simulink model "Simulink_Pendulum_Control_2019"  (R2019b)
settings: Solver=ode1  StartTime=0.0  StopTime=inf  FixedStep=0.002  RelTol=1e-3  EnableMultiTasking=on
PostLoadFcn:
  | qc_set_target_type(getConfigSet(bdroot, 'QUARC Default Target Configuration'));
values from neighbouring files (symbols this model uses):
  alpha_max = 15    [PolePlacement.m]
  theta_max = 45    [PolePlacement.m]
  voltage_max = 6    [PolePlacement.m]
undefined symbols (not defined in the file or in its folder): A_ob, B_ob, C_ob, D_ob, HIL, Ken_eta, Ken_x, qc_get_step_size, x0_ob
libraries: quarc_library x4, simulink_extras x1
settings Model: SimulationMode=external  ExtModeTrigDuration=5000  Creator=CFulford  LastModifiedBy=federicocorso
settings SolverCC: PositivePriorityOrder=on
settings DataIOCC: LimitDataPoints=on  SaveFormat=Array  SignalLoggingSaveFormat=ModelDataLogs  ReturnWorkspaceOutputs=off
settings OptimizationCC: ExpressionDepthLimit=2147483647  InitFltsAndDblsToZero=on  LifeSpan=inf
settings DebuggingCC: SaveWithParameterizedLinksMsg=none  UnderspecifiedInitializationDetection=Classic  MergeDetectMultiDrivingBlocksExec=none  SolverPrmCheckMsg=warning  MultiTaskDSMMsg=warning  MultiTaskCondExecSysMsg=none  FcnCallInpInsideContextMsg=warning  StateNameClashWarn=warning  SFUnexpectedBacktrackingDiag=warning  SFNoUnconditionalDefaultTransitionDiag=warning  SFExecutionAtInitializationDiag=none  ArithmeticOperatorsInVariantConditions=warning
settings HardwareCC: ProdBitPerPointer=32  ProdBitPerSizeT=32  ProdBitPerPtrDiffT=32  ProdLargestAtomicFloat=None  ProdIntDivRoundTo=Undefined  ProdEndianess=Unspecified  ProdWordSize=32  ProdHWDeviceType=32-bit Generic
settings ModelReferenceCC: PropagateSignalLabelsOutOfModel=off
settings SFSimCC: SimUseLocalCustomCode=off  CustomCodeUndefinedFunction=UseInterfaceOnly
settings RTWCC: Description=QUARC Win64 Target  SystemTargetFile=quarc_win64.tlc  TemplateMakefile=quarc_default_tmf  RTWUseLocalCustomCode=off
settings CodeAppCC: StateflowObjectComments=on
settings STFCustomTargetCC: TargetPreCompLibLocation=C:\PROGRA~3\QUARC\lib\2019b\win64\release  ConcurrentExecutionCompliant=on  CombineOutputUpdateFcns=on  CPPClassGenCompliant=on  SystemTargetFile=quarc_win64.tlc
settings GRTTargetCC: TargetPreCompLibLocation=C:\PROGRA~3\QUARC\lib\2019b\win64\release  TargetLangStandard=C89/C90 (ANSI)  ParMdlRefBuildCompliant=off  CompOptLevelCompliant=off  MatFileLogging=off  UseToolchainInfoCompliant=off  ExtMode=on  ExtModeMexFile=quarc_comm
settings ConfigComp: CovMetricSettings=dw  CovSaveCumulativeToWorkspaceVar=on  CovSaveSingleToWorkspaceVar=on  CovExternalEMLEnable=off  CovSFcnEnable=off

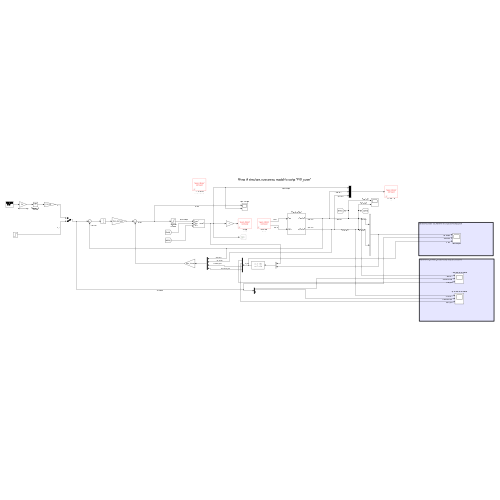
[thumbnail: Simulink's stored preview of the top-level diagram]
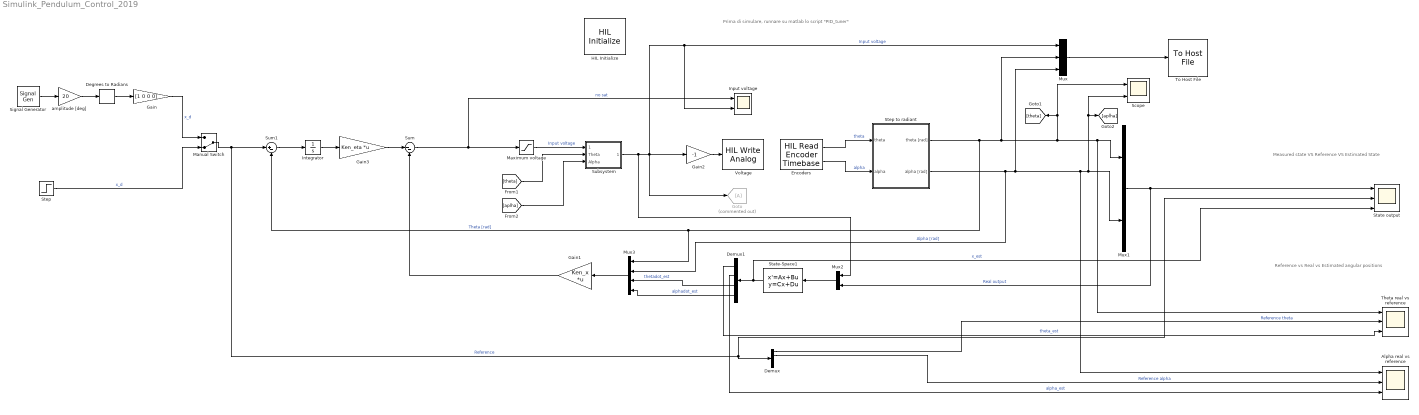
== system Simulink_Pendulum_Control_2019 ==
  note: Measured state VS Reference VS Estimated State
  note: Reference vs Real vs Estimated angular positions
  note: Prima di simulare, runnare su matlab lo script "PID_tuner"
  Alpha real vs reference : Scope  NumInputPorts=3
  Degrees to Radians : simulink_extras/Transformations/Degrees to Radians
  Demux : Demux
  Demux1 : Demux
  Encoders : quarc_library/Data Acquisition/Generic/Timebases/HIL Read Encoder Timebase  object_name=HIL-1  clock=0  channels=[0:1]  samples_in_buffer=max(ceil(1/qc_get_step_size), 1)  active=on  vector_output=off  data_type_mode=Inherit via back propagation  data_type=double
  Gain : Gain  Gain=[1 0 0 0]
  Gain1 : Gain  Gain=Ken_x  Multiplication=Matrix(K*u) (u vector)
  Gain2 : Gain  Gain=-1
  Gain3 : Gain  Gain=Ken_eta  Multiplication=Matrix(K*u) (u vector)
  Goto : Goto  Commented=on
  HIL Initialize : quarc_library/Data Acquisition/Generic/Configuration/HIL Initialize  Priority=-99  object_name=HIL-1  board_type=q2_usb  board_number=0  board_options=d0=digital;d1=digital;led=auto;update_rate=normal;decimation=1  exclusive=off  active=off  hardware_clocks=[0]  clock_modes=[]  initial_clock_frequencies=[]  set_clock_params_at_start=off  set_clock_params_at_switch_in=off  set_clock_frequencies_at_start=off  set_clock_frequencies_at_switch_in=off  analog_input_channels=[0:1]  analog_input_configurations=[]  analog_input_maximums=10  analog_input_minimums=-10  set_analog_input_params_at_start=on  set_analog_input_params_at_switch_in=off  analog_output_channels=[0:1]  analog_output_maximums=10  analog_output_minimums=-10  initial_analog_outputs=[0]  final_analog_outputs=[0]  watchdog_analog_outputs=0  set_analog_output_params_at_start=on  set_analog_output_params_at_switch_in=off  set_analog_outputs_at_start=on  set_analog_outputs_at_switch_in=off  set_analog_outputs_at_terminate=on  set_analog_outputs_at_switch_out=off  set_analog_outputs_on_watchdog=off  digital_input_channels=[]  digital_output_channels=[]  digital_output_configuration=[]  initial_digital_outputs=[1]  final_digital_outputs=[1]  watchdog_digital_outputs=[1]  set_digital_output_params_at_start=off  set_digital_output_params_at_switch_in=off  set_digital_outputs_at_start=on  set_digital_outputs_at_switch_in=off  set_digital_outputs_at_terminate=on  set_digital_outputs_at_switch_out=off  set_digital_outputs_on_watchdog=off  encoder_channels=[0:1]  quadrature=[4]  encoder_filter_frequency=[]  initial_encoder_counts=[0]  set_encoder_params_at_start=on  set_encoder_params_at_switch_in=off  set_encoder_counts_at_start=on  set_encoder_counts_at_switch_in=off  pwm_channels=[]  pwm_modes=[0]  pwm_frequency=1/0.020  pwm_configuration=[]  pwm_alignment=[]  pwm_polarity=[]  pwm_leading_deadband=[]  pwm_trailing_deadband=[]  initial_pwm_outputs=[0]  final_pwm_outputs=[0]  watchdog_pwm_outputs=[0]  set_pwm_params_at_start=on  set_pwm_params_at_switch_in=off  set_pwm_outputs_at_start=on  set_pwm_outputs_at_switch_in=off  set_pwm_outputs_at_terminate=on  set_pwm_outputs_at_switch_out=off  set_pwm_outputs_on_watchdog=off  other_output_channels=[]  initial_other_outputs=[]  final_other_outputs=[]  watchdog_other_outputs=[]  set_other_outputs_at_start=off  set_other_outputs_at_switch_in=off  set_other_outputs_at_terminate=off  set_other_outputs_at_switch_out=off  set_other_outputs_on_watchdog=off
  Input voltage : Scope  NumInputPorts=2
  Integrator : Integrator
  Manual Switch : ManualSwitch  CurrentSetting=0
  Maximum voltage : Saturate  UpperLimit=voltage_max  LowerLimit=-voltage_max
  Mux : Mux  Inputs=3
  Mux1 : Mux  Inputs=2
  Mux2 : Mux  Inputs=2
  Mux3 : Mux
  Scope : Scope  NumInputPorts=2
  Signal Generator : SignalGenerator  Frequency=0.1
  State output : Scope  NumInputPorts=3
  State-Space1 : StateSpace  A=A_ob  B=B_ob  C=C_ob  D=D_ob  InitialCondition=x0_ob
  Step : Step  Time=5  SampleTime=0
  Step to radiant : Subsystem
  Subsystem : Subsystem
  Sum : Sum  Inputs=|--
  Sum1 : Sum  Inputs=|+-
  Theta real vs reference : Scope  NumInputPorts=3
  To Host File : quarc_library/Sinks/To Host/To Host File  file_name=data_%{date}_%{time}.mat  variable_name=data_%{date}_%{time}  decimation=1  sample_time=-1  file_format=MAT-file v.5  options=No header or footer  append=off  final_file_name=data_28-Mar-2023_18-50-00.mat  bitrate=2000000
  Voltage : quarc_library/Data Acquisition/Generic/Immediate I//O/HIL Write Analog  object_name=HIL-1  channels=0  sample_time=-1  active=off  vector_input=off
  amplitude [deg] : Gain  Gain=20
  wires:
  Mux/1 -> To Host File/1
  Maximum voltage/1 -> Subsystem/1(Control)  "Input voltage"
  Gain2/1 -> Voltage/1
  Encoders/1 -> Step to radiant/1(theta)  "theta"
  Encoders/2 -> Step to radiant/2(alpha)  "alpha"
  Manual Switch/1 -> Sum1/1, State output/2, Demux/1  "Reference"
  amplitude [deg]/1 -> Degrees to Radians/1
  Signal Generator/1 -> amplitude [deg]/1
  Gain/1 -> Manual Switch/1  "x_d"
  Step/1 -> Manual Switch/2  "x_d"
  Degrees to Radians/1 -> Gain/1
  Sum/1 -> Input voltage/1, Maximum voltage/1  "no sat"
  Step to radiant/1(theta [rad]) -> Sum1/2, Mux3/1, Mux/2, Mux1/1, Theta real vs reference/1, Scope/1, [theta]  "Theta [rad]"
  Step to radiant/2(alpha [rad]) -> Mux3/2, Mux/3, Scope/2, [aplha], Mux1/2, Alpha real vs reference/1  "Alpha [rad]"
  Mux1/1 -> Mux2/2, State output/1  "Real output"
  Demux/2 -> Alpha real vs reference/2  "Reference alpha"
  Demux/1 -> Theta real vs reference/2  "Reference theta"
  [theta] -> Subsystem/2(Theta)
  [aplha] -> Subsystem/3(Alpha)
  Subsystem/1(control) -> Mux2/1, Goto/1, Mux/1, Input voltage/2, Gain2/1  "Input voltage"
  Mux2/1 -> State-Space1/1
  Mux3/1 -> Gain1/1
  State-Space1/1 -> State output/3, Demux1/1  "x_est"
  Demux1/3 -> Mux3/3  "thetadot_est"
  Demux1/4 -> Mux3/4  "alphadot_est"
  Demux1/1 -> Theta real vs reference/3  "theta_est"
  Demux1/2 -> Alpha real vs reference/3  "alpha_est"
  Gain3/1 -> Sum/1
  Integrator/1 -> Gain3/1
  Gain1/1 -> Sum/2
  Sum1/1 -> Integrator/1

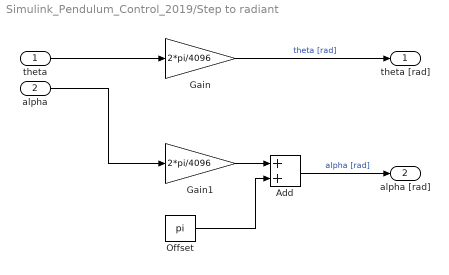
== system Simulink_Pendulum_Control_2019/Step to radiant ==
  theta : Inport
  alpha : Inport  Port=2
  Add : Sum
  Gain : Gain  Gain=2*pi/4096
  Gain1 : Gain  Gain=2*pi/4096
  Offset : Constant  Value=pi
  theta [rad] : Outport
  alpha [rad] : Outport  Port=2
  wires:
  Gain1/1 -> Add/1
  Gain/1 -> theta [rad]/1  "theta [rad]"
  Add/1 -> alpha [rad]/1  "alpha [rad]"
  Offset/1 -> Add/2
  theta/1 -> Gain/1
  alpha/1 -> Gain1/1

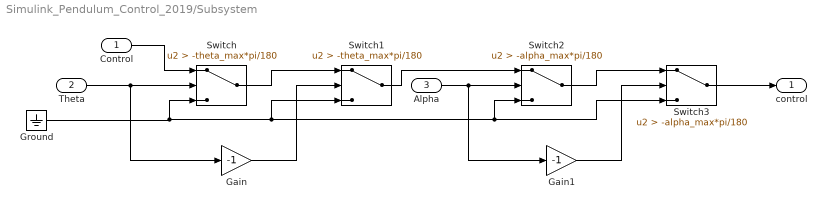
== system Simulink_Pendulum_Control_2019/Subsystem ==
  Control : Inport
  Theta : Inport  Port=2
  Alpha : Inport  Port=3
  Gain : Gain  Gain=-1
  Gain1 : Gain  Gain=-1
  Ground : Ground
  Switch : Switch  Criteria=u2 > Threshold  Threshold=-theta_max*pi/180
  Switch1 : Switch  Criteria=u2 > Threshold  Threshold=-theta_max*pi/180
  Switch2 : Switch  Criteria=u2 > Threshold  Threshold=-alpha_max*pi/180
  Switch3 : Switch  Criteria=u2 > Threshold  Threshold=-alpha_max*pi/180
  control : Outport
  wires:
  Gain/1 -> Switch1/2
  Theta/1 -> Gain/1, Switch/2
  Control/1 -> Switch/1
  Switch/1 -> Switch1/1
  Gain1/1 -> Switch3/2
  Switch1/1 -> Switch2/1
  Ground/1 -> Switch3/3, Switch2/3, Switch1/3, Switch/3
  Switch2/1 -> Switch3/1
  Alpha/1 -> Switch2/2, Gain1/1
  Switch3/1 -> control/1
